simulink model "gnc2_interface_unit_test"  (R2016b)
settings: Solver=FixedStepAuto  StartTime=0.0  StopTime=25  RelTol=1e-3
values from neighbouring files (symbols this model uses):
  GPS_epoch = sim_params.environment.sgp4.gps_time    [gnc2_interface_unit_test_init.m]
  hw_in = Jw * Om0    [gnc2_interface_unit_test_init.m]
  omega_cmd = [ 0.0; 0.0; 0.0 ]    [gnc2_interface_unit_test_init.m]
  omega_in = zeros(3,1)    [gnc2_interface_unit_test_init.m]
  quat_cmd = [ 1.0; 0.0; 0.0; 0.0 ]    [gnc2_interface_unit_test_init.m]
  quat_in = [ cosd(ang/2); sind(ang/2).*ax ]    [gnc2_interface_unit_test_init.m]
  sc_mode = 33    [gnc2_interface_unit_test_init.m]
  sI_unit = [ 1.0; 0.0; 0.0 ]    [gnc2_interface_unit_test_init.m]
libraries: GPS_time_lib x1, gnc2_interface_lib x1
settings Model: Creator=taylorreynolds  LastModifiedBy=Taylor

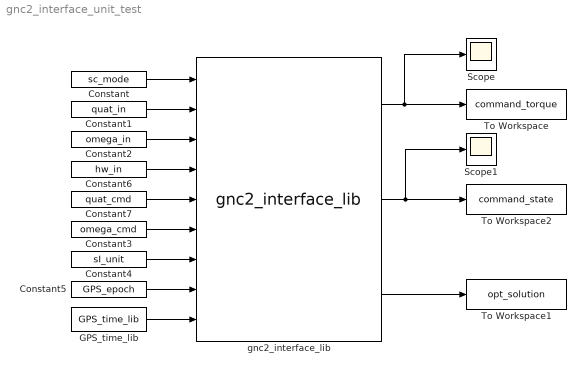
== system gnc2_interface_unit_test ==
  Constant : Constant  Value=sc_mode
  Constant1 : Constant  Value=quat_in
  Constant2 : Constant  Value=omega_in
  Constant3 : Constant  Value=omega_cmd
  Constant4 : Constant  Value=sI_unit
  Constant5 : Constant  Value=GPS_epoch
  Constant6 : Constant  Value=hw_in
  Constant7 : Constant  Value=quat_cmd
  GPS_time_lib : GPS_time_lib/GPS_time_lib
  Scope : Scope
  Scope1 : Scope
  To Workspace : ToWorkspace  VariableName=command_torque  SampleTime=-1
  To Workspace1 : ToWorkspace  VariableName=opt_solution  SampleTime=-1
  To Workspace2 : ToWorkspace  VariableName=command_state  SampleTime=-1
  gnc2_interface_lib : gnc2_interface_lib/gnc2_interface_lib
  wires:
  GPS_time_lib/1 -> gnc2_interface_lib/9
  Constant5/1 -> gnc2_interface_lib/8
  gnc2_interface_lib/1 -> To Workspace/1, Scope/1
  gnc2_interface_lib/3 -> To Workspace1/1
  Constant6/1 -> gnc2_interface_lib/4
  Constant7/1 -> gnc2_interface_lib/5
  Constant3/1 -> gnc2_interface_lib/6
  Constant4/1 -> gnc2_interface_lib/7
  Constant2/1 -> gnc2_interface_lib/3
  Constant1/1 -> gnc2_interface_lib/2
  Constant/1 -> gnc2_interface_lib/1
  gnc2_interface_lib/2 -> Scope1/1, To Workspace2/1
